simulink subsystem "SimulinkAveragedBuckConverterModel"  (R2022b)
settings: Solver=VariableStepAuto  StartTime=0.0  StopTime=10.0  RelTol=1e-3
undefined symbols (not defined in the file): C1, L1
settings Model: Creator=ykamatan  LastModifiedBy=ykamatan

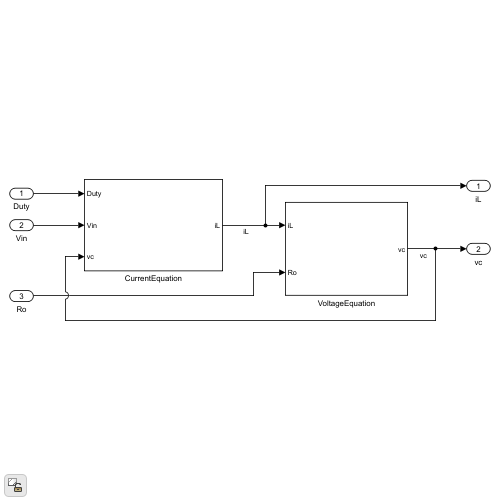
[thumbnail: Simulink's stored preview of the top-level diagram]
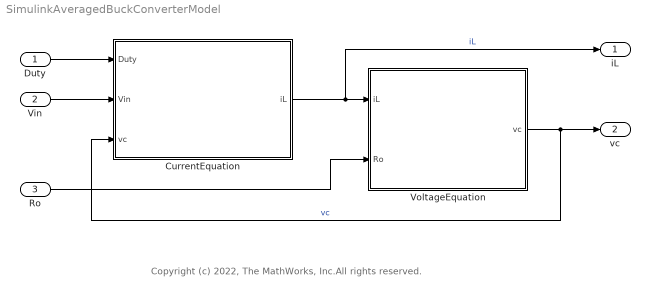
== system SimulinkAveragedBuckConverterModel ==
  note: Copyright (c) 2022, The MathWorks, Inc.All rights reserved.
  Duty : Inport
  Vin : Inport  Port=2
  Ro : Inport  Port=3
  CurrentEquation : Subsystem
  VoltageEquation : Subsystem
  iL : Outport
  vc : Outport  Port=2
  wires:
  CurrentEquation/1(iL) -> VoltageEquation/1(iL), iL/1  "iL"
  VoltageEquation/1(vc) -> CurrentEquation/3(vc), vc/1  "vc"
  Duty/1 -> CurrentEquation/1(Duty)
  Ro/1 -> VoltageEquation/2(Ro)
  Vin/1 -> CurrentEquation/2(Vin)

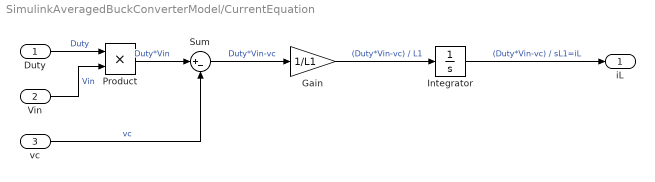
== system SimulinkAveragedBuckConverterModel/CurrentEquation ==
  Duty : Inport
  Vin : Inport  Port=2
  vc : Inport  Port=3
  Gain : Gain  Gain=1/L1
  Integrator : Integrator
  Product : Product
  Sum : Sum  Inputs=|+-
  iL : Outport
  wires:
  Sum/1 -> Gain/1  "Duty*Vin-vc"
  vc/1 -> Sum/2  "vc"
  Product/1 -> Sum/1  "Duty*Vin"
  Vin/1 -> Product/2  "Vin"
  Duty/1 -> Product/1  "Duty"
  Gain/1 -> Integrator/1  "(Duty*Vin-vc) / L1"
  Integrator/1 -> iL/1  "(Duty*Vin-vc) / sL1=iL"

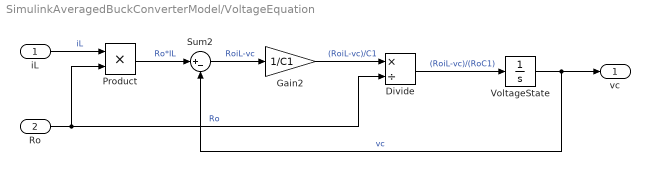
== system SimulinkAveragedBuckConverterModel/VoltageEquation ==
  iL : Inport
  Ro : Inport  Port=2
  Divide : Product  Inputs=*/
  Gain2 : Gain  Gain=1/C1
  Product : Product
  Sum2 : Sum  Inputs=|+-
  VoltageState : Integrator
  vc : Outport
  wires:
  Divide/1 -> VoltageState/1  "(RoiL-vc)/(RoC1)"
  Ro/1 -> Product/2, Divide/2  "Ro"
  Product/1 -> Sum2/1  "Ro*IL"
  iL/1 -> Product/1  "iL"
  Sum2/1 -> Gain2/1  "RoiL-vc"
  Gain2/1 -> Divide/1  "(RoiL-vc)/C1"
  VoltageState/1 -> vc/1, Sum2/2  "vc"
